simulink model "sonmodel"  (R2023a)
settings: Solver=VariableStepAuto  StartTime=0.0  StopTime=100  RelTol=1e-3
values from neighbouring files (symbols this model uses):
  b = 1    [KATSAYI.m]    (also in hiz.m = 0.1; kat.m = 0.1; matlab.mat; untitled.m = 0.1)
  B1 = 1    [KATSAYI.m]    (also in hiz.m; kat.m; matlab.mat; untitled.m)
  B2 = 1    [KATSAYI.m]    (also in hiz.m; kat.m; matlab.mat; untitled.m)
  J = 1    [KATSAYI.m]    (also in hiz.m = 0.01; kat.m = 0.01; matlab.mat; untitled.m = 0.01)
  J1 = 1    [KATSAYI.m]    (also in hiz.m = 0.1; kat.m = 0.1; matlab.mat; untitled.m)
  J2 = 1    [KATSAYI.m]    (also in hiz.m = 0.1; kat.m = 0.1; matlab.mat; untitled.m)
  K = 1    [KATSAYI.m]    (also in hiz.m = 0.01; kat.m = 0.01; matlab.mat; untitled.m = 0.01)
  K1 = 1    [KATSAYI.m]    (also in hiz.m = 100; kat.m = 100; matlab.mat; untitled.m)
  Kd = 18.6251550360015    (= 18.625155036)    [kat.m]
  Ki = 12.6968787117754    (= 12.6968787118)    [kat.m]
  Kp = 43.8419795726236    (= 43.8419795726)    [kat.m]
  L = 1    [KATSAYI.m]    (also in hiz.m = 0.5; kat.m = 0.5; matlab.mat; untitled.m = 0.5)
  R = 1    [KATSAYI.m]    (also in hiz.m; kat.m; matlab.mat; untitled.m)
libraries: fl_lib x7, nesl_utility x7, sdl_lib x2, slpidlib x2, ee_lib x1
settings Model: Creator=monster  LastModifiedBy=monster
settings DebuggingCC: ParameterPrecisionLossMsg=none

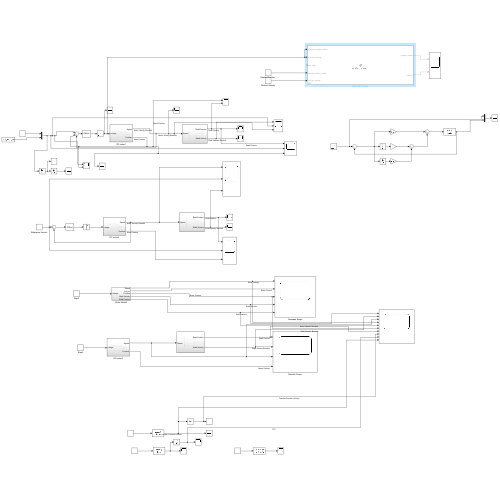
[thumbnail: Simulink's stored preview of the top-level diagram]
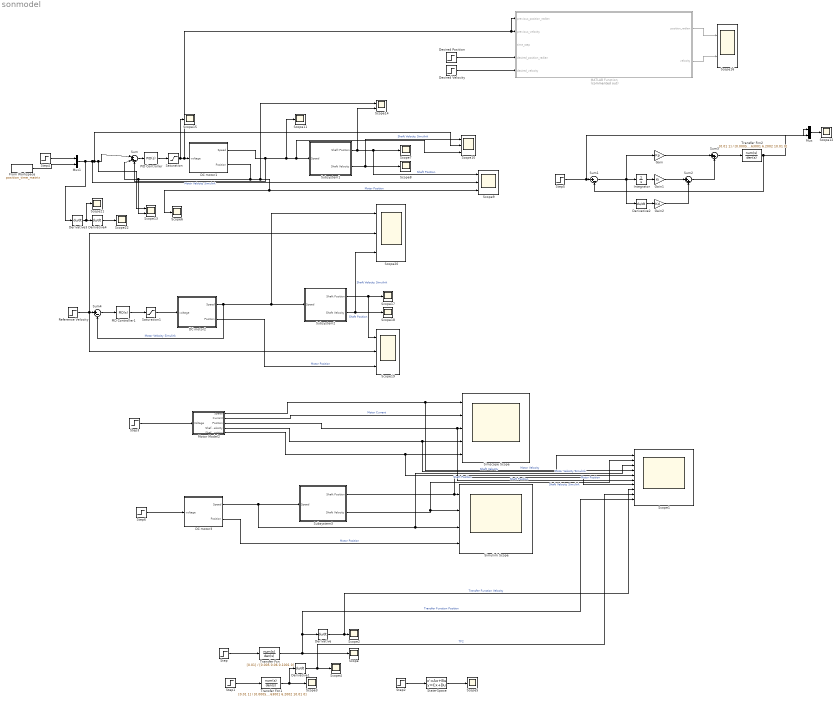
== system sonmodel ==
  DC motor1 : Subsystem
  DC motor2 : Subsystem
  DC motor3 : Subsystem
  Derivative{,1..4} (5 alike) : Derivative
  "Desired Position " : Step  After=50  SampleTime=0
  Desired Velocity : Step  After=5  SampleTime=0
  From Workspace : FromWorkspace  VariableName=position_time_matrix
  Gain : Gain  Gain=Kp
  Gain1 : Gain  Gain=Ki
  Gain2 : Gain  Gain=Kd
  Integrator : Integrator
  MATLAB Function : MATLAB Function  Commented=on  TreatAsAtomicUnit=on
  Motor Model2 : Subsystem
  Mux : Mux  Inputs=2
  Mux1 : Mux  Inputs=2
  PID Controller : slpidlib/PID Controller  Controller=PID  Form=Parallel  TimeDomain=Continuous-time  UseExternalTs=off  SampleTime=-1  IntegratorMethod=Forward Euler  FilterMethod=Forward Euler  ControllerParametersSource=internal  P=34.1898064142988  I=9.2752929302529  UseKiTs=off  D=19.9937403530455  N=405.494741877744  UseFilter=on  TunerSelectOption=Transfer Function Based (PID Tuner App)  InitialConditionSource=internal  InitialConditionForIntegrator=0  InitialConditionForFilter=0  DifferentiatorICPrevScaledInput=0  ExternalReset=none  TrackingMode=off  Kt=1  LimitOutput=off  SatLimitsSource=internal  UpperSaturationLimit=10  LowerSaturationLimit=-10  LinearizeAsGain=on  AntiWindupMode=none  Kb=1  LimitIntegrator=off  UpperIntegratorSaturationLimit=10  LowerIntegratorSaturationLimit=-10  POutMin=[]  POutMax=[]  IOutMin=[]  IOutMax=[]  DOutMin=[]  DOutMax=[]  NOutMin=[]  NOutMax=[]  SumOutMin=[]  SumOutMax=[]  SaturationOutMin=[]  SaturationOutMax=[]  PParamMin=[]  PParamMax=[]  IParamMin=[]  IParamMax=[]  DParamMin=[]  DParamMax=[]  NParamMin=[]  NParamMax=[]  KbParamMin=[]  KbParamMax=[]  KtParamMin=[]  KtParamMax=[]  KbOutMin=[]  KbOutMax=[]  KtOutMin=[]  KtOutMax=[]  IntegratorOutMin=[]  IntegratorOutMax=[]  FilterOutMin=[]  FilterOutMax=[]  SumI1OutMin=[]  SumI1OutMax=[]  SumI2OutMin=[]  SumI2OutMax=[]  SumI3OutMin=[]  SumI3OutMax=[]  SumI4OutMin=[]  SumI4OutMax=[]  SumDOutMin=[]  SumDOutMax=[]  DifferentiatorOutMin=[]  DifferentiatorOutMax=[]  FilterDiffOutCoefMin=[]  FilterDiffOutCoefMax=[]  ReciprocalOutMin=[]  ReciprocalOutMax=[]  SumDenOutMin=[]  SumDenOutMax=[]  SumNumOutMin=[]  SumNumOutMax=[]  DivideOutMin=[]  DivideOutMax=[]  UdiffTsProdOutMin=[]  UdiffTsProdOutMax=[]  NTsProdOutMin=[]  NTsProdOutMax=[]  UintegralTsProdOutMin=[]  UintegralTsProdOutMax=[]  UngainTsProdOutMin=[]  UngainTsProdOutMax=[]  ClampingZeroOutDataTypeStr=Inherit: Inherit via back propagation  ClampingZeroOutMin=[]  ClampingZeroOutMax=[]  FilterDenConstantOutDataTypeStr=Inherit: Inherit via back propagation  FilterDenConstantOutMin=[]  FilterDenConstantOutMax=[]  PCopyOutDataTypeStr=Inherit: Inherit via back propagation  PCopyOutMin=[]  PCopyOutMax=[]  NCopyOutDataTypeStr=Inherit: Inherit via back propagation  NCopyOutMin=[]  NCopyOutMax=[]  IntegratorContinuousStateAttributes=''  IntegratorStateMustResolveToSignalObject=off  IntegratorRTWStateStorageClass=Auto  FilterContinuousStateAttributes=''  FilterStateMustResolveToSignalObject=off  FilterRTWStateStorageClass=Auto  ParallelPVariant=InternalParameters  IdealPVariant=Disabled  IVariant=InternalParameters  DVariant=InternalParameters  IntegratorVariant=Continuous  SatVariant=Disabled  AWVariant=Passthrough  PCopyVariant=Disabled  TRVariant=Disabled  FdbkBlocksVariant=Forward  IdealPFdbkVariant=Disabled  SatFdbkVariant=Disabled  DerivativeFilterVariant=ContFilter  NVariant=InternalParameters  NCopyVariant=Disabled  FilterICVariant=InternalICsFilter  IntegratorICVariant=InternalICs  ExternalResetVariant=Disabled  TRSumVariant=Passthrough  SumFdbkVariant=Disabled  SumVariant=Sum_PID  TsampFilterVariant=InternalTs  TsampNgainVariant=Passthrough  TsampIntegralVariant=Disabled_SignalSpec  ExternalSaturationOutDataTypeStr=Inherit: Same as second input
  PID Controller1 : slpidlib/PID Controller  Controller=PID  Form=Parallel  TimeDomain=Continuous-time  UseExternalTs=off  SampleTime=-1  IntegratorMethod=Forward Euler  FilterMethod=Forward Euler  ControllerParametersSource=internal  P=43.8419795726236  I=12.6968787117754  UseKiTs=off  D=18.6251550360015  N=405.494741877744  UseFilter=on  TunerSelectOption=Transfer Function Based (PID Tuner App)  InitialConditionSource=internal  InitialConditionForIntegrator=0  InitialConditionForFilter=0  DifferentiatorICPrevScaledInput=0  ExternalReset=none  TrackingMode=off  Kt=1  LimitOutput=off  SatLimitsSource=internal  UpperSaturationLimit=10  LowerSaturationLimit=-10  LinearizeAsGain=on  AntiWindupMode=none  Kb=1  LimitIntegrator=off  UpperIntegratorSaturationLimit=10  LowerIntegratorSaturationLimit=-10  POutMin=[]  POutMax=[]  IOutMin=[]  IOutMax=[]  DOutMin=[]  DOutMax=[]  NOutMin=[]  NOutMax=[]  SumOutMin=[]  SumOutMax=[]  SaturationOutMin=[]  SaturationOutMax=[]  PParamMin=[]  PParamMax=[]  IParamMin=[]  IParamMax=[]  DParamMin=[]  DParamMax=[]  NParamMin=[]  NParamMax=[]  KbParamMin=[]  KbParamMax=[]  KtParamMin=[]  KtParamMax=[]  KbOutMin=[]  KbOutMax=[]  KtOutMin=[]  KtOutMax=[]  IntegratorOutMin=[]  IntegratorOutMax=[]  FilterOutMin=[]  FilterOutMax=[]  SumI1OutMin=[]  SumI1OutMax=[]  SumI2OutMin=[]  SumI2OutMax=[]  SumI3OutMin=[]  SumI3OutMax=[]  SumI4OutMin=[]  SumI4OutMax=[]  SumDOutMin=[]  SumDOutMax=[]  DifferentiatorOutMin=[]  DifferentiatorOutMax=[]  FilterDiffOutCoefMin=[]  FilterDiffOutCoefMax=[]  ReciprocalOutMin=[]  ReciprocalOutMax=[]  SumDenOutMin=[]  SumDenOutMax=[]  SumNumOutMin=[]  SumNumOutMax=[]  DivideOutMin=[]  DivideOutMax=[]  UdiffTsProdOutMin=[]  UdiffTsProdOutMax=[]  NTsProdOutMin=[]  NTsProdOutMax=[]  UintegralTsProdOutMin=[]  UintegralTsProdOutMax=[]  UngainTsProdOutMin=[]  UngainTsProdOutMax=[]  ClampingZeroOutDataTypeStr=Inherit: Inherit via back propagation  ClampingZeroOutMin=[]  ClampingZeroOutMax=[]  FilterDenConstantOutDataTypeStr=Inherit: Inherit via back propagation  FilterDenConstantOutMin=[]  FilterDenConstantOutMax=[]  PCopyOutDataTypeStr=Inherit: Inherit via back propagation  PCopyOutMin=[]  PCopyOutMax=[]  NCopyOutDataTypeStr=Inherit: Inherit via back propagation  NCopyOutMin=[]  NCopyOutMax=[]  IntegratorContinuousStateAttributes=''  IntegratorStateMustResolveToSignalObject=off  IntegratorRTWStateStorageClass=Auto  FilterContinuousStateAttributes=''  FilterStateMustResolveToSignalObject=off  FilterRTWStateStorageClass=Auto  ParallelPVariant=InternalParameters  IdealPVariant=Disabled  IVariant=InternalParameters  DVariant=InternalParameters  IntegratorVariant=Continuous  SatVariant=Disabled  AWVariant=Passthrough  PCopyVariant=Disabled  TRVariant=Disabled  FdbkBlocksVariant=Forward  IdealPFdbkVariant=Disabled  SatFdbkVariant=Disabled  DerivativeFilterVariant=ContFilter  NVariant=InternalParameters  NCopyVariant=Disabled  FilterICVariant=InternalICsFilter  IntegratorICVariant=InternalICs  ExternalResetVariant=Disabled  TRSumVariant=Passthrough  SumFdbkVariant=Disabled  SumVariant=Sum_PID  TsampFilterVariant=InternalTs  TsampNgainVariant=Passthrough  TsampIntegralVariant=Disabled_SignalSpec  ExternalSaturationOutDataTypeStr=Inherit: Same as second input
  Reference Velocity : Step  SampleTime=0
  Saturation : Saturate  UpperLimit=50  LowerLimit=-50
  Saturation1 : Saturate  UpperLimit=255  LowerLimit=-255
  Scope{,2..8,11..12,15,17..18,21..22} (15 alike) : Scope
  Scope1 : Scope  NumInputPorts=10
  Scope{9..10,19..20} (4 alike) : Scope  NumInputPorts=3
  Scope13 : Scope  NumInputPorts=2
  Scope14 : Scope  NumInputPorts=2
  Scope16 : Scope  NumInputPorts=2
  Simscape Scope : Scope  NumInputPorts=5
  Simulink Scope : Scope  NumInputPorts=4
  State-Space : StateSpace  A=[-32 -1260 -12400 -20020 0; 1 0 0 0 0; 0 1 0 0 0; 0 0 1 0 0; 0 0 0 1 0]  B=[1; 0; 0; 0; 0]  C=[0 0 0 20 2000]  D=[0]  InitialCondition=[0;0;0;0;0]
  Step{,1..4,6} (6 alike) : Step  After=5  SampleTime=0
  Step5 : Step  SampleTime=0
  Subsystem1 : Subsystem
  Subsystem2 : Subsystem
  Subsystem3 : Subsystem
  Sum : Sum  Inputs=|+--
  Sum1 : Sum  Inputs=|+-
  Sum2 : Sum  Inputs=|++
  Sum3 : Sum  Inputs=|++
  Sum4 : Sum  Inputs=|+-
  Transfer Fcn : TransferFcn  Numerator=[0.01]  Denominator=[0.005 0.06 0.1001 0]  ContinuousStateAttributes='position'
  Transfer Fcn1 : TransferFcn  Numerator=[0.01 1]  Denominator=[0.0005 0.016 0.63001 6.2002 10.01 0]
  Transfer Fcn2 : TransferFcn  Numerator=[0.01 1]  Denominator=[0.0005 0.016 0.63001 6.2002 10.01 0]
  wires:
  Motor Model2/4(Shaft Velocity) -> Scope1/1, Simscape Scope/4  "Shaft Velocity"
  Motor Model2/1(Speed) -> Scope1/4, Simscape Scope/1  "Motor Velocity"
  Motor Model2/3(Position) -> Scope1/6, Simscape Scope/3  "Motor Position"
  Motor Model2/2(Current) -> Simscape Scope/2  "Motor Current"
  Subsystem3/1(Shaft Position) -> Scope1/7, Simulink Scope/1  "Shaft Position"
  Step6/1 -> DC motor3/1(voltage)
  DC motor3/1(Speed) -> Scope1/3, Simulink Scope/3, Subsystem3/1(Speed)  "Motor Velocity Simulink"
  Motor Model2/5(Shaft Position) -> Scope1/5, Simscape Scope/5  "Shaft Position"
  Subsystem3/2(Shaft Velocity) -> Scope1/2, Simulink Scope/2  "Shaft Velocity Simulink"
  DC motor3/2(Position) -> Simulink Scope/4  "Motor Position"
  Derivative/1 -> Scope1/8, Scope2/1  "Transfer Function Velocity"
  Step/1 -> Transfer Fcn/1
  Transfer Fcn/1 -> Scope1/10, Derivative/1, Scope/1  "Transfer Function Position"
  Step1/1 -> Transfer Fcn1/1
  Transfer Fcn1/1 -> Derivative1/1, Scope3/1
  Derivative1/1 -> Scope1/9, Scope4/1  "TF2"
  Step2/1 -> State-Space/1
  State-Space/1 -> Scope5/1
  Step3/1 -> Motor Model2/1(Voltage)
  DC motor1/1(Speed) -> Sum/3, Scope11/1, Scope10/3, Subsystem1/1(Speed)  "Motor Velocity Simulink"
  DC motor1/2(Position) -> Scope13/2, Sum/2, Scope6/1, Scope9/3, Scope14/1  "Motor Position"
  Subsystem1/1(Shaft Position) -> Scope14/2, Scope9/1, Scope7/1  "Shaft Position"
  Subsystem1/2(Shaft Velocity) -> Scope10/1, Scope8/1  "Shaft Velocity Simulink"
  PID Controller/1 -> Saturation/1
  Step4/1 -> Mux1/1
  Sum/1 -> PID Controller/1
  Step5/1 -> Mux/1, Sum1/1
  Sum1/1 -> Derivative2/1, Gain/1, Integrator/1
  Integrator/1 -> Gain1/1
  Derivative2/1 -> Gain2/1
  Gain2/1 -> Sum2/2
  Gain1/1 -> Sum2/1
  Gain/1 -> Sum3/1
  Sum2/1 -> Sum3/2
  Sum3/1 -> Transfer Fcn2/1
  Transfer Fcn2/1 -> Sum1/2, Mux/2
  Mux/1 -> Scope12/1
  Saturation/1 -> Scope15/1, MATLAB Function/1(previous_position_radian), MATLAB Function/2(previous_velocity), DC motor1/1(voltage)
  MATLAB Function/1(position_radian) -> Scope16/1
  MATLAB Function/2(velocity) -> Scope16/2
  DC motor2/1(Speed) -> Scope20/1, Subsystem2/1(Speed), Sum4/2  "Motor Velocity Simulink"
  Subsystem2/1(Shaft Position) -> Scope19/1, Scope17/1  "Shaft Position"
  Subsystem2/2(Shaft Velocity) -> Scope20/3, Scope18/1  "Shaft Velocity Simulink"
  Saturation1/1 -> DC motor2/1(voltage)
  PID Controller1/1 -> Saturation1/1
  Sum4/1 -> PID Controller1/1
  Reference Velocity/1 -> Scope20/2, Scope19/2, Sum4/1
  DC motor2/2(Position) -> Scope19/3  "Motor Position"
  "Desired Position "/1 -> MATLAB Function/4(desired_position_radian)
  Desired Velocity/1 -> MATLAB Function/5(desired_velocity)
  Derivative3/1 -> Scope21/1, Derivative4/1
  Derivative4/1 -> Scope22/1
  From Workspace/1 -> Mux1/2
  Mux1/1 -> Derivative3/1, Scope9/2, Scope10/2, Scope13/1, Sum/1

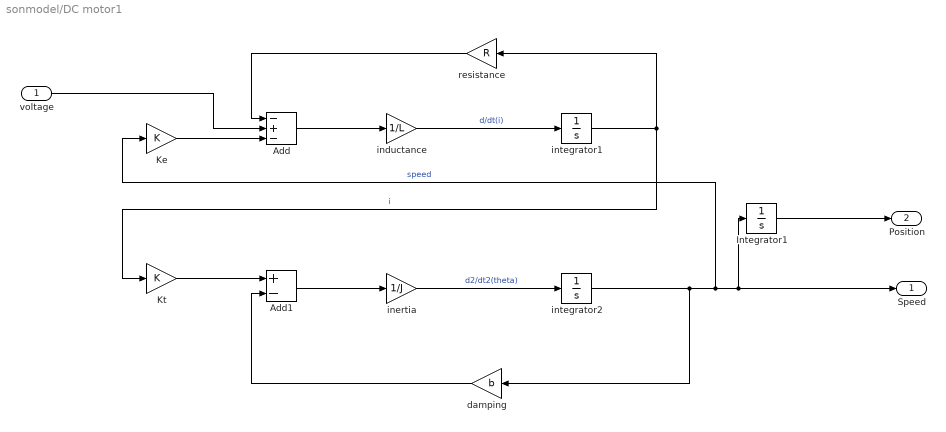
== system sonmodel/DC motor1 ==
  voltage : Inport
  Add : Sum  Inputs=-+-
  Add1 : Sum  Inputs=+-
  Integrator1 : Integrator
  Ke : Gain  Gain=K
  Kt : Gain  Gain=K
  damping : Gain  Gain=b
  "inductance " : Gain  Gain=1/L
  inertia : Gain  Gain=1/J
  integrator1 : Integrator
  integrator2 : Integrator
  resistance : Gain  Gain=R
  Speed : Outport
  Position : Outport  Port=2
  wires:
  damping/1 -> Add1/2
  Add1/1 -> inertia/1
  Kt/1 -> Add1/1
  integrator1/1 -> resistance/1, Kt/1  "i"
  Add/1 -> "inductance "/1
  voltage/1 -> Add/2
  resistance/1 -> Add/1
  inertia/1 -> integrator2/1  "d2/dt2(theta)"
  integrator2/1 -> damping/1, Integrator1/1, Speed/1, Ke/1  "speed"
  Ke/1 -> Add/3
  "inductance "/1 -> integrator1/1  "d/dt(i)"
  Integrator1/1 -> Position/1

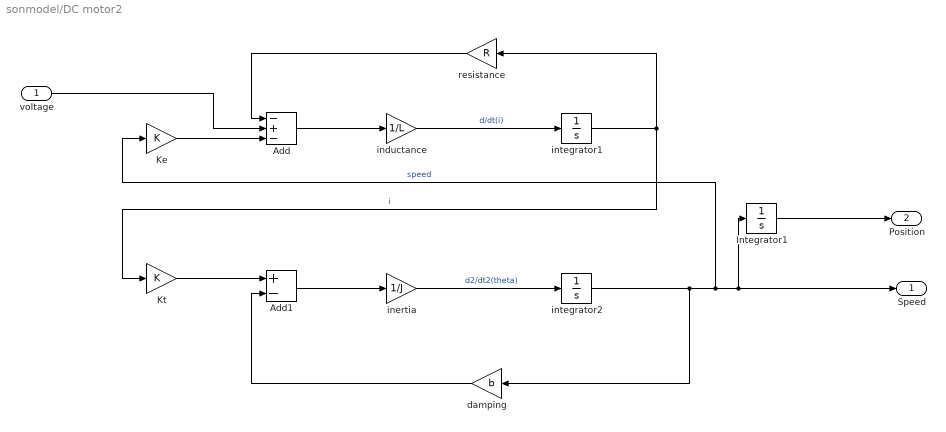
== system sonmodel/DC motor2 ==
  voltage : Inport
  Add : Sum  Inputs=-+-
  Add1 : Sum  Inputs=+-
  Integrator1 : Integrator
  Ke : Gain  Gain=K
  Kt : Gain  Gain=K
  damping : Gain  Gain=b
  "inductance " : Gain  Gain=1/L
  inertia : Gain  Gain=1/J
  integrator1 : Integrator
  integrator2 : Integrator
  resistance : Gain  Gain=R
  Speed : Outport
  Position : Outport  Port=2
  wires:
  damping/1 -> Add1/2
  Add1/1 -> inertia/1
  Kt/1 -> Add1/1
  integrator1/1 -> resistance/1, Kt/1  "i"
  Add/1 -> "inductance "/1
  voltage/1 -> Add/2
  resistance/1 -> Add/1
  inertia/1 -> integrator2/1  "d2/dt2(theta)"
  integrator2/1 -> damping/1, Integrator1/1, Speed/1, Ke/1  "speed"
  Ke/1 -> Add/3
  "inductance "/1 -> integrator1/1  "d/dt(i)"
  Integrator1/1 -> Position/1

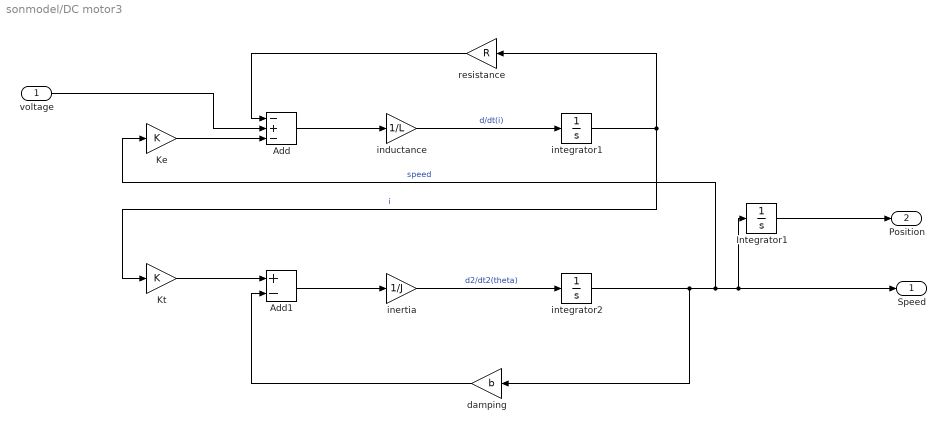
== system sonmodel/DC motor3 ==
  voltage : Inport
  Add : Sum  Inputs=-+-
  Add1 : Sum  Inputs=+-
  Integrator1 : Integrator
  Ke : Gain  Gain=K
  Kt : Gain  Gain=K
  damping : Gain  Gain=b
  "inductance " : Gain  Gain=1/L
  inertia : Gain  Gain=1/J
  integrator1 : Integrator
  integrator2 : Integrator
  resistance : Gain  Gain=R
  Speed : Outport
  Position : Outport  Port=2
  wires:
  damping/1 -> Add1/2
  Add1/1 -> inertia/1
  Kt/1 -> Add1/1
  integrator1/1 -> resistance/1, Kt/1  "i"
  Add/1 -> "inductance "/1
  voltage/1 -> Add/2
  resistance/1 -> Add/1
  inertia/1 -> integrator2/1  "d2/dt2(theta)"
  integrator2/1 -> damping/1, Integrator1/1, Speed/1, Ke/1  "speed"
  Ke/1 -> Add/3
  "inductance "/1 -> integrator1/1  "d/dt(i)"
  Integrator1/1 -> Position/1

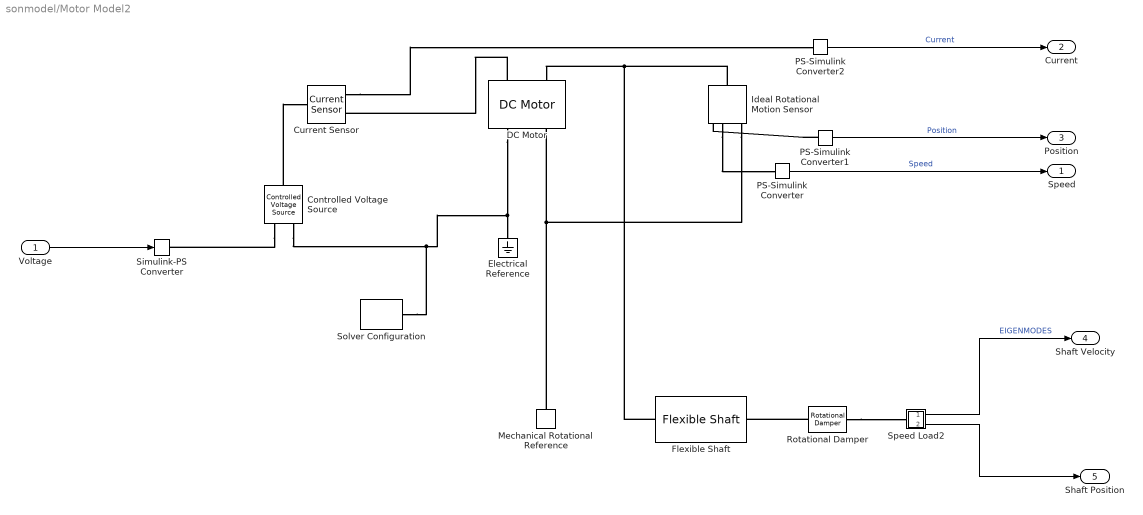
== system sonmodel/Motor Model2 ==
  Voltage : Inport
  Controlled Voltage Source : fl_lib/Electrical/Electrical Sources/Controlled Voltage Source
  Current Sensor : fl_lib/Electrical/Electrical Sensors/Current Sensor
  DC Motor : ee_lib/Electromechanical/Brushed Motors/DC Motor  field_option=ee.enum.field_option.pm  Rf=100 Ohm  Lf=1 H  Laf=0.15 H  If0=0 A  parameterization=ee.enum.dcparam_option.circuit_param  Ra=1 Ohm  La=0.5 H  emf_or_torque=ee.enum.emf_or_torque.kv  Kv=0.01 V/(rad/s)  Ki=6.876e-4 N*m/A  T_stall=0.24e-3 N*m  w_max=19100 rpm  w_rated=15000 rpm  P_rated=0.08 W  V_rated=1.5 V  lam_param=ee.enum.lam_param.damping  i_noload=0 A  V_i_noload=1.5 V  J=0.01 kg*m^2  lam=0.1 N*m/(rad/s)  speed0=0 rpm  enable_fault_armature=simscape.enum.onoff.off  rev_faulted=1 / 3  G_faulted_armature=1e-5 S  fault_trigger_armature=ee.enum.faults.faultTrigger.temporal  t_fault_armature=1 s  max_permissible_current_armature=inf A  t_fail_on_current_armature=1 s  enable_fault_field=simscape.enum.onoff.off  G_faulted_field=1e-5 S  fault_trigger_field=ee.enum.faults.faultTrigger.temporal  t_fault_field=1 s  max_permissible_current_field=inf A  t_fail_on_current_field=1 s  fault_action=simscape.enum.assert.action.none  alpha=3.93e-3 1/K  Tmeas=25 degC  thermal_mass=100 J/K  initial_temperature=25 degC
  Electrical Reference : fl_lib/Electrical/Electrical Elements/Electrical Reference
  Flexible Shaft : sdl_lib/Couplings & Drives/Flexible Shaft  modelTorsion=true  modelTransverse=false  n_segments=1  parameterization=sdl.enum.shaftParameterization.StiffnessInertia  length=1 m  lengths=[1, .5, .25] m  shaft_stiffness=100 N*m/rad  shaft_inertia=0.1 kg*m^2  shaft_stiffnesses=[400000, 200000, 100000] N*m/rad  shaft_inertias=[.025, .02, .015] kg*m^2  eiIN=5e5 Pa*m^4  rhoaIN=19 kg/m  eiINs=[600000, 500000, 400000] Pa*m^4  rhoaINs=[20, 19, 18] kg/m  density=7.8e3 kg/m^3  shear_modulus=7.93e9 Pa  elastic_modulus=200e9 Pa  shaft_construction=sdl.enum.shaftConstruction.solid  diameter_outer=0.075 m  diameter_inner=0.05 m  diameter_outers=[.085, .075, .065] m  diameter_inners=[.055, .05, .045] m  damping_ratio=1  mu_visc_BF=[0, 0] N*m*s/rad  mu_visc=[0, 0] N*m*s/rad  initial_deflection=0 rad  initial_velocity=0 rpm  num_supports=sdl.enum.num_supports.two  z_support=[0, 1] m  boundaryB1=sdl.enum.shaftSupport.clamp  DrotB1_row=[1000, 1000] N*m*s/rad  DtransB1_row=[20000, -44000, -44000, 350000] N*s/m  DtransB1_w_mat=[20000, -44000, -44000, 350000; 10000, -25000, -25000, 140000; 5000, -10000, -10000, 20000] N*s/m  KrotB1_row=[10000, 10000] N*m/rad  KtransB1_row=[1000000, -200000, -300000, 5000000] N/m  KtransB1_w_mat=[1000000, -600000, -3500000, 8000000; 1000000, -200000, -3000000, 5000000; 1000000, -50000, -2500000, 3000000] N/m  boundaryI1=sdl.enum.shaftSupport.clamp  DrotI1_row=[1000, 1000] N*m*s/rad  DtransI1_row=[20000, -44000, -44000, 350000] N*s/m  DtransI1_w_mat=[20000, -44000, -44000, 350000; 10000, -25000, -25000, 140000; 5000, -10000, -10000, 20000] N*s/m  KrotI1_row=[10000, 10000] N*m/rad  KtransI1_row=[1000000, -200000, -300000, 5000000] N/m  KtransI1_w_mat=[1000000, -600000, -3500000, 8000000; 1000000, -200000, -3000000, 5000000; 1000000, -50000, -2500000, 3000000] N/m  boundaryI2=sdl.enum.shaftSupport.clamp  DrotI2_row=[1000, 1000] N*m*s/rad  DtransI2_row=[20000, -44000, -44000, 350000] N*s/m  DtransI2_w_mat=[20000, -44000, -44000, 350000; 10000, -25000, -25000, 140000; 5000, -10000, -10000, 20000] N*s/m  KrotI2_row=[10000, 10000] N*m/rad  KtransI2_row=[1000000, -200000, -300000, 5000000] N/m  KtransI2_w_mat=[1000000, -600000, -3500000, 8000000; 1000000, -200000, -3000000, 5000000; 1000000, -50000, -2500000, 3000000] N/m  boundaryF1=sdl.enum.shaftSupport.clamp  DrotF1_row=[1000, 1000] N*m*s/rad  DtransF1_row=[20000, -44000, -44000, 350000] N*s/m  DtransF1_w_mat=[20000, -44000, -44000, 350000; 10000, -25000, -25000, 140000; 5000, -10000, -10000, 20000] N*s/m  KrotF1_row=[10000, 10000] N*m/rad  KtransF1_row=[1000000, -200000, -300000, 5000000] N/m  KtransF1_w_mat=[1000000, -600000, -3500000, 8000000; 1000000, -200000, -3000000, 5000000; 1000000, -50000, -2500000, 3000000] N/m  bearing_speed=[200, 500, 1500] rpm  alpha=10 1/s  beta=1e-8 s  noDisk=sdl.enum.shaftDisks.none  zDisk=0.5 m  mDiskIN=2 kg  IdDiskIN=0.025 kg*m^2  IpDiskIN=0.050 kg*m^2  enable_static_unbalance=true  offsetMR=[.01, .01] kg*m  offsetMR_initialAngleIN=[0, pi] rad  offsetMassLocation=[.33, .67] m  enable_external_force=false  externalForce=[1, 2] N  externalForceHarmonic=[.5, 2]  externalLoadAngle=[pi / 2, 3 * pi / 4] rad  zExternalLoad=[.25, .75] m  AnalysisMethod=sdl.enum.bendingAnalysisMethod.LumpedMass  ModeInputMethod=sdl.enum.modeInputMethod.SimscapeDetermined  numModesIn=6  mode_speed_dependency=sdl.enum.mode_speed_dependency.Static  OmegaNom=5000 rpm  wMax=1e8 rpm  dz=0.01 m  userMode_w=[280, 644, 615, 1285] rad/s  userMode_w_mat=[257, 780, 580, 1560; 280, 644, 615, 1285; 294, 513, 636, 1020] rad/s  userMode_z=[0, .1, .2, .3, .4, .5, .6, .7, .8, .9, 1] m  userMode_shapeX=[.1648, .0086, -.2759, .0162; .1671, .0093, -.2231, .0133; .1691, .01, -.1689, .0102; .1707, .0105, -.1135, .007; .1717, .0108, -.057, .0035; .1721, .0109, 0, 0; .1717, .0108, .057, -.0035; .1707, .0105, .1135, -.007; .1691, .01, .1689, -.0102; .1671, .0093, .2231, -.0133; .1648, .0086, .2759, -.0162]  userMode_shapeX_mat=cat(3, [.1842, .0134, -.3072, .0272; .1863, .0152, -.2482, .0226; .1882, .0169, -.1878, .0176; .1897, .0182, -.1261, .0121; .1906, .019, -.0634, .0062; .191, .0193, 0, 0; .1906, .019, .0634, -.0062; .1897, .0182, .1261, -.0121; .1882, .0169, .1878, -.0176; .1863, .0152, .2482, -.0226; .1842, .0134, .3072, -.0272], [.1648, .0086, -.2759, .0162; .1671, .0093, -.2231, .0133; .1691, .01, -.1689, .0102; .1707, .0105, -.1135, .007; .1717, .0108, -.057, .0035; .1721, .0109, 0, 0; .1717, .0108, .057, -.0035; .1707, .0105, .1135, -.007; .1691, .01, .1689, -.0102; .1671, .0093, .2231, -.0133; .1648, .0086, .2759, -.0162], [.1291, .0046, -.2166, .0082; .131, .0048, -.1751, .0067; .1327, .005, -.1327, .0051; .1341, .0052, -.0891, .0035; .135, .0053, -.0448, .0017; .1353, .0053, 0, 0; .135, .0053, .0448, -.0017; .1341, .0052, .0891, -.0035; .1327, .005, .1327, -.0051; .131, .0048, .1751, -.0067; .1291, .0046, .2166, -.0082])  userMode_shapeY=[.1193, -.1784, -.1997, -.3348; .1209, -.1933, -.1615, -.2751; .1224, -.2068, -.1223, -.2119; .1235, -.2176, -.0821, -.1445; .1243, -.2245, -.0413, -.0734; .1246, -.2269, 0, 0; .1243, -.2245, .0413, .0734; .1235, -.2176, .0821, .1445; .1224, -.2068, .1223, .2119; .1209, -.1933, .1615, .2751; .1193, -.1784, .1997, .3348]  userMode_shapeY_mat=cat(3, [.0885, -.1625, -.1475, -.3301; .0895, -.1847, -.1192, -.2745; .0904, -.2048, -.0902, -.2141; .0911, -.2209, -.0606, -.1475; .0916, -.2313, -.0304, -.0754; .0917, -.2349, 0, 0; .0916, -.2313, .0304, .0754; .0911, -.2209, .0606, .1475; .0904, -.2048, .0902, .2141; .0895, -.1847, .1192, .2745; .0885, -.1625, .1475, .3301], [.1193, -.1784, -.1997, -.3348; .1209, -.1933, -.1615, -.2751; .1224, -.2068, -.1223, -.2119; .1235, -.2176, -.0821, -.1445; .1243, -.2245, -.0413, -.0734; .1246, -.2269, 0, 0; .1243, -.2245, .0413, .0734; .1235, -.2176, .0821, .1445; .1224, -.2068, .1223, .2119; .1209, -.1933, .1615, .2751; .1193, -.1784, .1997, .3348], [.1566, -.1901, -.2628, -.3377; .1589, -.1994, -.2125, -.2753; .161, -.2079, -.1609, -.2103; .1627, -.2146, -.1081, -.1424; .1638, -.219, -.0544, -.0719; .1642, -.2205, 0, 0; .1638, -.219, .0544, .0719; .1627, -.2146, .1081, .1424; .161, -.2079, .1609, .2103; .1589, -.1994, .2125, .2753; .1566, -.1901, .2628, .3377])  eta_lumped_nominal=1  etaDer_lumped_nominal=1  eta_modal_nominal=1  etaDer_modal_nominal=1
      settings: InternalSimscapePortConfiguration="{\"Bottom\":[],\"Left\":[{\"id\":\"B\",\"label\":\"B\",\"type\":\"foundation.mechanical.rotational.rotational\"}],\"Right\":[{\"id\":\"F\",\"label\":\"F\",\"type\":\"foundation.mechanical.rotational.rotational\"}],\"Top\":[]}"
  Ideal Rotational Motion Sensor : fl_lib/Mechanical/Mechanical Sensors/Ideal Rotational Motion Sensor  reference=foundation.enum.MeasurementReference.difference  acceleration_port=true  velocity_port=true  position_port=true  wrap_angle=true  offset=0 rad
      settings: InternalSimscapePortConfiguration="{\"Bottom\":[],\"Left\":[{\"id\":\"R\",\"label\":\"R\",\"type\":\"foundation.mechanical.rotational.rotational\"}],\"Right\":[{\"id\":\"C\",\"label\":\"C\",\"type\":\"foundation.mechanical.rotational.rotational\"},{\"id\":\"alpha\",\"label\":\"α\",\"type\":\"output\"},{\"id\":\"W\",\"label\":\"W\",\"type\":\"output\"},{\"id\":\"A\",\"label\":\"A\",\"type\":\"output\"}],\"Top\":[]}"
  Mechanical Rotational Reference : fl_lib/Mechanical/Rotational Elements/Mechanical Rotational Reference
  PS-Simulink Converter : nesl_utility/PS-Simulink Converter  PhysicalDomain=network_engine_domain  SubClassName=ps_output  LeftPortType=input  RightPortType=output  PseudoPeriodic=off  Frequencies=[]  VectorFormat=inherit  Unit=rad/s  AffineConversion=off
  PS-Simulink Converter1 : nesl_utility/PS-Simulink Converter  PhysicalDomain=network_engine_domain  SubClassName=ps_output  LeftPortType=input  RightPortType=output  PseudoPeriodic=off  Frequencies=[]  VectorFormat=inherit  Unit=rad  AffineConversion=off
  PS-Simulink Converter2 : nesl_utility/PS-Simulink Converter  PhysicalDomain=network_engine_domain  SubClassName=ps_output  LeftPortType=input  RightPortType=output  PseudoPeriodic=off  Frequencies=[]  VectorFormat=inherit  Unit=A  AffineConversion=off
  Rotational Damper : sdl_lib/Couplings & Drives/Springs & Dampers/Rotational Damper  D=1 N*m*s/rad  enable_faults=simscape.enum.onoff.off  b_fault=100 N*m*s/rad  temporal_fault=simscape.enum.onoff.off  fault_time=5 s  shock_fault=simscape.enum.onoff.off  acceleration_limit=100 rad/s^2  shock_limit=1  report_fault=simscape.enum.assert.action.none  thermal_port=simscape.enum.thermaleffects.omit  thermal_mass=50 kJ/K  temperature_specify=off  temperature_priority=High  temperature=300 K  temperature_nominal_specify=off  temperature_nominal_unit=K  temperature_nominal_value=1
  Simulink-PS Converter : nesl_utility/Simulink-PS Converter  PhysicalDomain=network_engine_domain  SubClassName=ps_input  LeftPortType=input  RightPortType=output  PseudoPeriodic=off  Frequencies=[]  NoiseDistribution=none  NoiseParameters=[]  Unit=V  AffineConversion=off  FilteringAndDerivatives=provide  SimscapeFilterOrder=1  InputFilterTimeConstant=0.001  UdotUserProvided=0
  Solver Configuration : nesl_utility/Solver Configuration  PhysicalDomain=network_engine_domain  SubClassName=solver  LeftPortType=input  RightPortType=generic  Tones=[]  Harmonics=[]  SimulateNoise=off  Profile=off  UseLocalSampling=off  EnableSwitchedLinearOptims=on  FrequencyDomain=off  UseCCode=off  RelTol=0.001  AbsTol=0.001  MinStep=1e-09  ToWorkspace=off  RevertToSquareIcSolve=off  NumHomotopyIterations=100  PhasorMode=off  PhasorModeNumHarmonics=1  ConsistencySolver=NEWTON_XTOL_AFTER_FTOL  IndexReductionMethod=DerivativeReplacement  DoDC=off  ResidualTolerance=1e-09  ConsistencyTolSource=GLOBAL  ConsistencyAbsTol=0.001  ConsistencyRelTol=0.001  ConsistencyTolFactor=0.001  UseLocalSolver=off  LocalSolverChoice=NE_BACKWARD_EULER_ADVANCER  ResolveIndetEquations=on  FunctionEvalNumThread=1  LocalSolverSampleTime=0.001  DoFixedCost=off  MaxNonlinIter=3  MaxModeIter=2  ComputeImpulses=off  ImpulseIterations=2  LinearAlgebra=auto  LinearAlgebraNumThread=0  EquationFormulation=NE_TIME_EF  DelaysMemoryBudget=1024  AutomaticFiltering=on  FilteringTimeConstant=0.001  PartitionStorageMethod=AS_NEEDED  PartitionMemoryBudget=1024  PartitionMethod=ROBUST
  Speed Load2 : Subsystem
      mask Display: disp('w')
  Speed : Outport
  Current : Outport  Port=2
  Position : Outport  Port=3
  Shaft Velocity : Outport  Port=4
  Shaft Position : Outport  Port=5
  wires:
  PS-Simulink Converter1/1 -> Position/1  "Position"
  PS-Simulink Converter2/1 -> Current/1  "Current"
  Voltage/1 -> Simulink-PS Converter/1
  PS-Simulink Converter/1 -> Speed/1  "Speed"
  Speed Load2/1(w) -> Shaft Velocity/1  "EIGENMODES"
  Speed Load2/2(Out1) -> Shaft Position/1
  connections:
  Controlled Voltage Source/RConn2 -- Solver Configuration/RConn1 -- DC Motor/RConn1 -- Electrical Reference/LConn1
  Controlled Voltage Source/RConn1 -- Simulink-PS Converter/RConn1
  Current Sensor/RConn1 -- PS-Simulink Converter2/LConn1
  Mechanical Rotational Reference/LConn1 -- Ideal Rotational Motion Sensor/RConn1 -- DC Motor/RConn2
  Ideal Rotational Motion Sensor/LConn1 -- Flexible Shaft/LConn1 -- DC Motor/LConn2
  DC Motor/LConn1 -- Current Sensor/RConn2
  Controlled Voltage Source/LConn1 -- Current Sensor/LConn1
  Ideal Rotational Motion Sensor/RConn3 -- PS-Simulink Converter/LConn1
  PS-Simulink Converter1/LConn1 -- Ideal Rotational Motion Sensor/RConn4
  Rotational Damper/LConn1 -- Flexible Shaft/RConn1
  Rotational Damper/RConn1 -- Speed Load2/LConn1

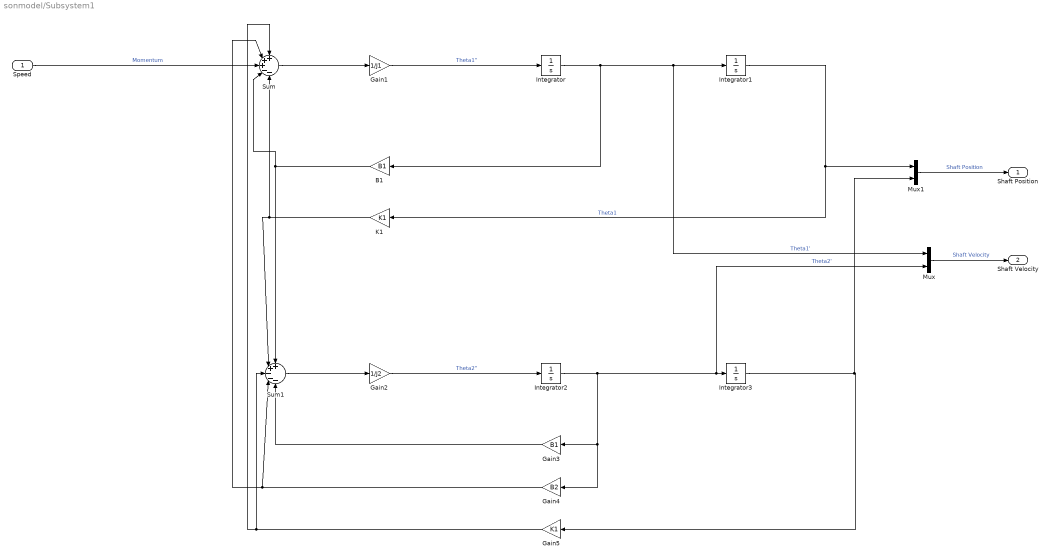
== system sonmodel/Subsystem1 ==
  Speed : Inport
  B1 : Gain  Gain=B1
  Gain1 : Gain  Gain=1/J1
  Gain2 : Gain  Gain=1/J2
  Gain3 : Gain  Gain=B1
  Gain4 : Gain  Gain=B2
  Gain5 : Gain  Gain=K1
  Integrator{,1..3} (4 alike) : Integrator
  K1 : Gain  Gain=K1
  Mux : Mux  Inputs=2
  Mux1 : Mux  Inputs=2
  Sum : Sum  Inputs=+++--
  Sum1 : Sum  Inputs=++---
  Shaft Position : Outport
  Shaft Velocity : Outport  Port=2
  wires:
  Gain5/1 -> Sum1/3, Sum/1
  Integrator3/1 -> Gain5/1, Mux1/2
  Gain4/1 -> Sum/2, Sum1/4
  Gain3/1 -> Sum1/5
  Integrator2/1 -> Mux/2, Integrator3/1, Gain3/1, Gain4/1  "Theta2'"
  Gain2/1 -> Integrator2/1  "Theta2''"
  Sum1/1 -> Gain2/1
  K1/1 -> Sum1/2, Sum/5
  Integrator1/1 -> Mux1/1, K1/1  "Theta1"
  B1/1 -> Sum/4, Sum1/1
  Integrator/1 -> Mux/1, Integrator1/1, B1/1  "Theta1'"
  Gain1/1 -> Integrator/1  "Theta1''"
  Speed/1 -> Sum/3  "Momentum"
  Sum/1 -> Gain1/1
  Mux1/1 -> Shaft Position/1  "Shaft Position"
  Mux/1 -> Shaft Velocity/1  "Shaft Velocity"

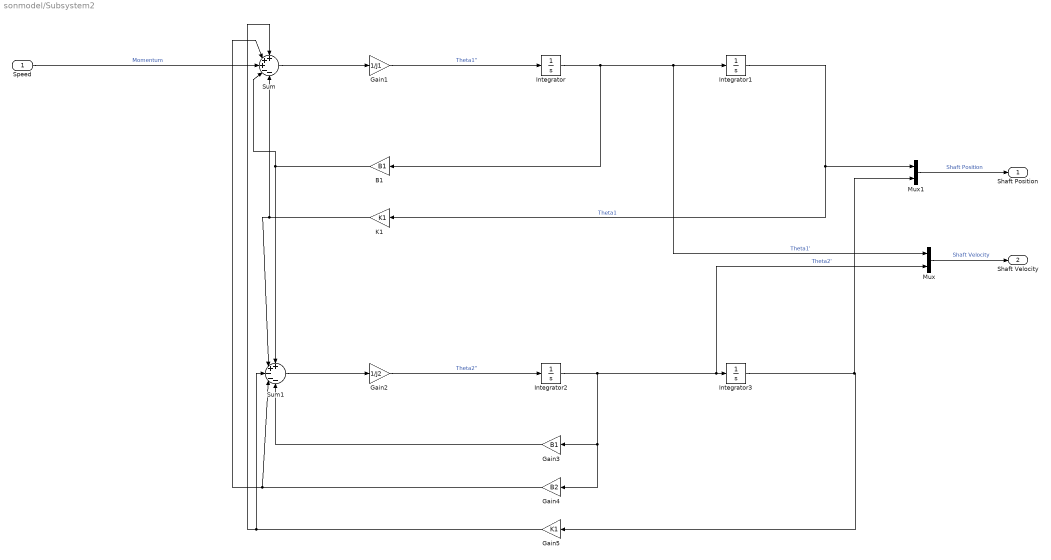
== system sonmodel/Subsystem2 ==
  Speed : Inport
  B1 : Gain  Gain=B1
  Gain1 : Gain  Gain=1/J1
  Gain2 : Gain  Gain=1/J2
  Gain3 : Gain  Gain=B1
  Gain4 : Gain  Gain=B2
  Gain5 : Gain  Gain=K1
  Integrator{,1..3} (4 alike) : Integrator
  K1 : Gain  Gain=K1
  Mux : Mux  Inputs=2
  Mux1 : Mux  Inputs=2
  Sum : Sum  Inputs=+++--
  Sum1 : Sum  Inputs=++---
  Shaft Position : Outport
  Shaft Velocity : Outport  Port=2
  wires:
  Gain5/1 -> Sum1/3, Sum/1
  Integrator3/1 -> Gain5/1, Mux1/2
  Gain4/1 -> Sum/2, Sum1/4
  Gain3/1 -> Sum1/5
  Integrator2/1 -> Mux/2, Integrator3/1, Gain3/1, Gain4/1  "Theta2'"
  Gain2/1 -> Integrator2/1  "Theta2''"
  Sum1/1 -> Gain2/1
  K1/1 -> Sum1/2, Sum/5
  Integrator1/1 -> Mux1/1, K1/1  "Theta1"
  B1/1 -> Sum/4, Sum1/1
  Integrator/1 -> Mux/1, Integrator1/1, B1/1  "Theta1'"
  Gain1/1 -> Integrator/1  "Theta1''"
  Speed/1 -> Sum/3  "Momentum"
  Sum/1 -> Gain1/1
  Mux1/1 -> Shaft Position/1  "Shaft Position"
  Mux/1 -> Shaft Velocity/1  "Shaft Velocity"

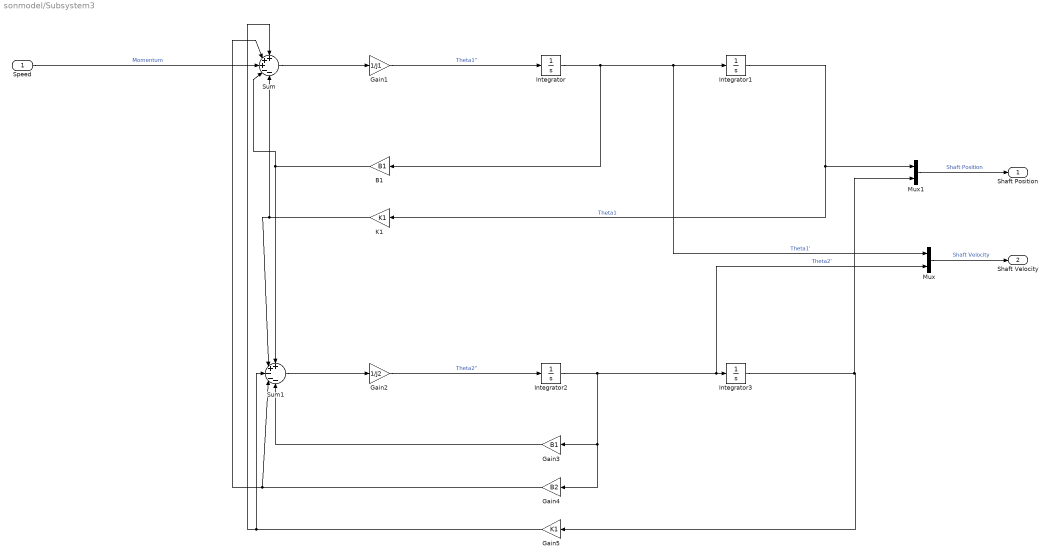
== system sonmodel/Subsystem3 ==
  Speed : Inport
  B1 : Gain  Gain=B1
  Gain1 : Gain  Gain=1/J1
  Gain2 : Gain  Gain=1/J2
  Gain3 : Gain  Gain=B1
  Gain4 : Gain  Gain=B2
  Gain5 : Gain  Gain=K1
  Integrator{,1..3} (4 alike) : Integrator
  K1 : Gain  Gain=K1
  Mux : Mux  Inputs=2
  Mux1 : Mux  Inputs=2
  Sum : Sum  Inputs=+++--
  Sum1 : Sum  Inputs=++---
  Shaft Position : Outport
  Shaft Velocity : Outport  Port=2
  wires:
  Gain5/1 -> Sum1/3, Sum/1
  Integrator3/1 -> Gain5/1, Mux1/2
  Gain4/1 -> Sum/2, Sum1/4
  Gain3/1 -> Sum1/5
  Integrator2/1 -> Mux/2, Integrator3/1, Gain3/1, Gain4/1  "Theta2'"
  Gain2/1 -> Integrator2/1  "Theta2''"
  Sum1/1 -> Gain2/1
  K1/1 -> Sum1/2, Sum/5
  Integrator1/1 -> Mux1/1, K1/1  "Theta1"
  B1/1 -> Sum/4, Sum1/1
  Integrator/1 -> Mux/1, Integrator1/1, B1/1  "Theta1'"
  Gain1/1 -> Integrator/1  "Theta1''"
  Speed/1 -> Sum/3  "Momentum"
  Sum/1 -> Gain1/1
  Mux1/1 -> Shaft Position/1  "Shaft Position"
  Mux/1 -> Shaft Velocity/1  "Shaft Velocity"

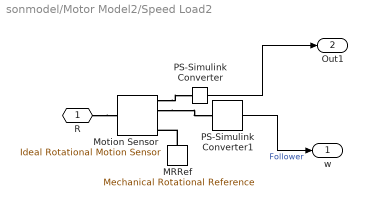
== system sonmodel/Motor Model2/Speed Load2 ==
  MRRef : fl_lib/Mechanical/Rotational Elements/Mechanical Rotational Reference
  Motion Sensor : fl_lib/Mechanical/Mechanical Sensors/Ideal Rotational Motion Sensor  reference=foundation.enum.MeasurementReference.difference  acceleration_port=true  velocity_port=true  position_port=true  wrap_angle=true  offset=0 rad
      settings: InternalSimscapePortConfiguration="{\"Bottom\":[],\"Left\":[{\"id\":\"R\",\"label\":\"R\",\"type\":\"foundation.mechanical.rotational.rotational\"}],\"Right\":[{\"id\":\"C\",\"label\":\"C\",\"type\":\"foundation.mechanical.rotational.rotational\"},{\"id\":\"alpha\",\"label\":\"α\",\"type\":\"output\"},{\"id\":\"W\",\"label\":\"W\",\"type\":\"output\"},{\"id\":\"A\",\"label\":\"A\",\"type\":\"output\"}],\"Top\":[]}"
  PS-Simulink Converter : nesl_utility/PS-Simulink Converter  PhysicalDomain=network_engine_domain  SubClassName=ps_output  LeftPortType=input  RightPortType=output  PseudoPeriodic=off  Frequencies=[]  VectorFormat=inherit  Unit=inherit  AffineConversion=off
  PS-Simulink Converter1 : nesl_utility/PS-Simulink Converter  PhysicalDomain=network_engine_domain  SubClassName=ps_output  LeftPortType=input  RightPortType=output  PseudoPeriodic=off  Frequencies=[]  VectorFormat=1-D array  Unit=rad/s  AffineConversion=off
  R : PMIOPort  Side=Left
  w : Outport  VectorParamsAs1DForOutWhenUnconnected=off
  Out1 : Outport  Port=2
  wires:
  PS-Simulink Converter1/1 -> w/1  "Follower"
  PS-Simulink Converter/1 -> Out1/1
  connections:
  R/RConn1 -- Motion Sensor/LConn1
  MRRef/LConn1 -- Motion Sensor/RConn1
  Motion Sensor/RConn3 -- PS-Simulink Converter1/LConn1
  Motion Sensor/RConn4 -- PS-Simulink Converter/LConn1

== matlab function sonmodel/MATLAB Function ==
  data: previous_position_radian input; position_radian output; previous_velocity input; time_step input; desired_position_radian input; desired_velocity input; velocity output
function [position_radian, velocity] = simulate_encoder(previous_position_radian, previous_velocity, time_step, desired_position_radian, desired_velocity)
    % Simülasyon parametreleri
    encoder_resolution = 1000; % Kodlayıcı çözünürlüğü (pulse/sayı)
    max_velocity = 10; % Maksimum hız (rad/s)

    % Pozisyonun radyan cinsinden hesaplanması
    previous_position_pulse = previous_position_radian * encoder_resolution / (2 * pi);

    % Hız kontrolü: Motorun istenen hıza ulaşması
    if desired_position_radian > previous_position_radian
        motor_velocity = min(desired_velocity, max_velocity); % İleri hareket için
    else
        motor_velocity = max(-desired_velocity, -max_velocity); % Geri hareket için
    end

    % Motorun yeni pozisyonu ve hızı
    position_pulse = previous_position_pulse + previous_velocity * time_step;
    velocity = motor_velocity;

    % Kodlayıcı sinyallerinin simülasyonu
    encoder_pulse = motor_velocity / (2 * pi) * encoder_resolution; % Kodlayıcı sinyali (pulse/s)
    position_pulse = mod(position_pulse + encoder_pulse, encoder_resolution); % Pozisyon döngüsü

    % Pozisyonun 0 ile encoder_resolution arasında tutulması
    if position_pulse < 0
        position_pulse = position_pulse + encoder_resolution;
    end

    % Güncellenmiş pozisyonun radyan cinsinden hesaplanması
    position_radian = position_pulse * (2 * pi) / encoder_resolution;
end
